simulink model "part1"  (R2025a)
settings: Solver=ode45  StartTime=0.0  StopTime=30.0  RelTol=1e-3
settings Model: Creator=z.yin  LastModifiedBy=z.yin

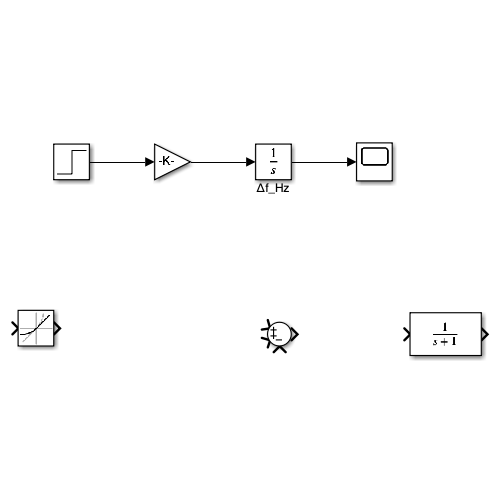
[thumbnail: Simulink's stored preview of the top-level diagram]
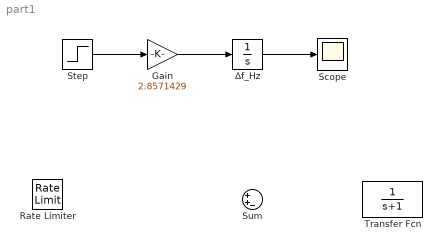
== system part1 ==
  Gain : Gain  Gain=2.8571429
  Rate Limiter : RateLimiter  SampleTimeMode=inherited
  Scope : Scope
  Step : Step  Time=0  After=0.05  SampleTime=0
  Sum : Sum  Inputs=|++-
  Transfer Fcn : TransferFcn  Denominator=[1 1]
  Δf_Hz : Integrator
  wires:
  Step/1 -> Gain/1
  Gain/1 -> Δf_Hz/1
  Δf_Hz/1 -> Scope/1
